simulink model "calcAcceleration"  (R2019a)
settings: Solver=FixedStepAuto  StartTime=0  StopTime=inf  FixedStep=1e-3  MaxStep=1e-3  RelTol=1e-3
values from neighbouring files (symbols this model uses):
  init =     [course_data_0_1m.mat]
libraries: simulink x1
settings Model: Creator=Frieder Uerlings  LastModifiedBy=Frieder Uerlings
settings SolverCC: ZeroCrossControl=DisableAll  AlgebraicLoopSolver=LineSearch

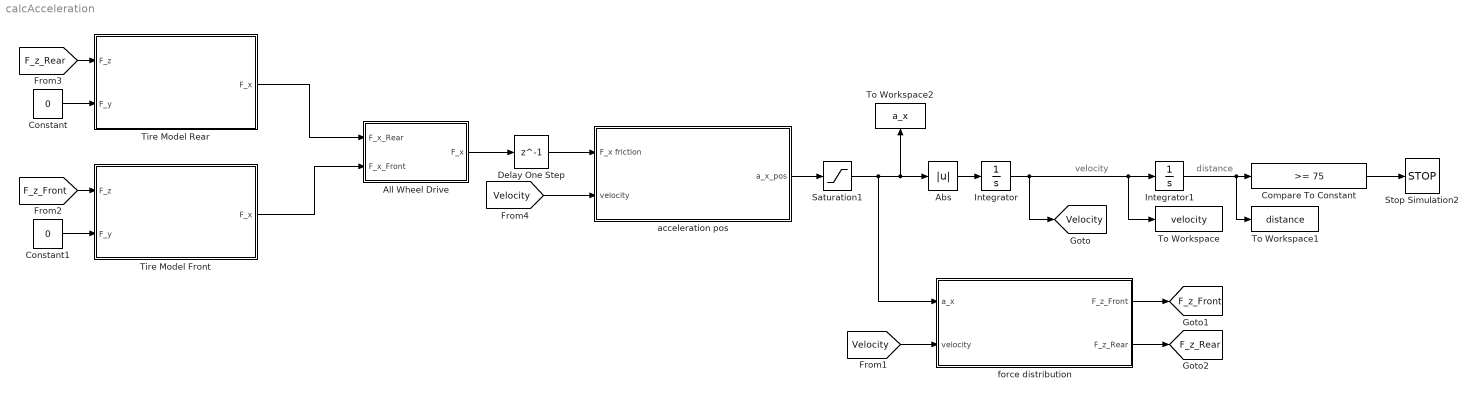
== system calcAcceleration ==
  note: distance
  note: velocity
  Abs : Abs
  All Wheel Drive : Subsystem
  Compare To Constant : simulink/Logic and Bit Operations/Compare To Constant  relop=>=  const=75  OutDataTypeStr=boolean
  Constant : Constant  Value=0
  Constant1 : Constant  Value=0
  Delay One Step : Delay  DelayLength=1
  Integrator : Integrator  InitialCondition=1/inf
  Integrator1 : Integrator
  Saturation1 : Saturate  UpperLimit=inf  LowerLimit=0  ZeroCross=off
  Stop Simulation2 : Stop
  Tire Model Front : Subsystem
  Tire Model Rear : Subsystem
  To Workspace : ToWorkspace  VariableName=velocity  SampleTime=-1
  To Workspace1 : ToWorkspace  VariableName=distance  SampleTime=-1
  To Workspace2 : ToWorkspace  VariableName=a_x  SampleTime=-1
  "acceleration pos " : Subsystem
  force distribution : Subsystem
  tag scope: F_z_Front=global, F_z_Rear=global, Velocity=global
  wires:
  Compare To Constant/1 -> Stop Simulation2/1
  Integrator/1 -> [Velocity], To Workspace/1, Integrator1/1
  Saturation1/1 -> Abs/1, To Workspace2/1, force distribution/1("a_x ")
  Integrator1/1 -> To Workspace1/1, Compare To Constant/1
  [Velocity] -> force distribution/2("velocity ")
  force distribution/1(F_z_Front) -> [F_z_Front]
  force distribution/2("F_z_Rear ") -> [F_z_Rear]
  [F_z_Front] -> Tire Model Front/1(F_z)
  [F_z_Rear] -> Tire Model Rear/1(F_z)
  Delay One Step/1 -> "acceleration pos "/1(F_x friction)
  "acceleration pos "/1("a_x_pos ") -> Saturation1/1
  Tire Model Front/1(F_x) -> All Wheel Drive/2(F_x_Front)
  Tire Model Rear/1(F_x) -> All Wheel Drive/1(F_x_Rear)
  [Velocity] -> "acceleration pos "/2(velocity)
  Abs/1 -> Integrator/1
  All Wheel Drive/1(F_x) -> Delay One Step/1
  Constant/1 -> Tire Model Rear/2(F_y)
  Constant1/1 -> Tire Model Front/2(F_y)

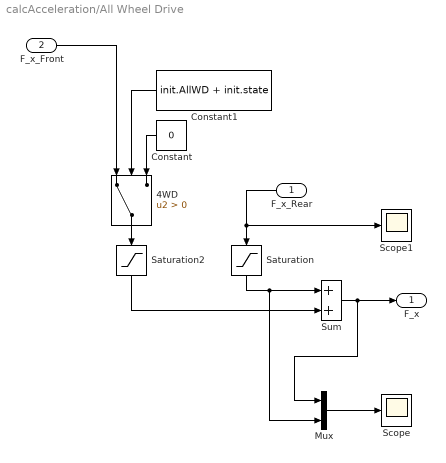
== system calcAcceleration/All Wheel Drive ==
  F_x_Rear : Inport
  F_x_Front : Inport  Port=2
  4WD : Switch  Criteria=u2 > Threshold
  Constant : Constant  Value=0
  Constant1 : Constant  Value=init.AllWD + init.state
  Mux : Mux  Inputs=2
  Saturation : Saturate  UpperLimit=inf  LowerLimit=0
  Saturation2 : Saturate  UpperLimit=inf  LowerLimit=0
  Scope : Scope
  Scope1 : Scope
  Sum : Sum
  F_x : Outport
  wires:
  Constant1/1 -> 4WD/2
  F_x_Rear/1 -> Scope1/1, Saturation/1
  4WD/1 -> Saturation2/1
  Constant/1 -> 4WD/3
  F_x_Front/1 -> 4WD/1
  Saturation/1 -> Mux/2, Sum/1
  Saturation2/1 -> Sum/2
  Sum/1 -> Mux/1, F_x/1
  Mux/1 -> Scope/1

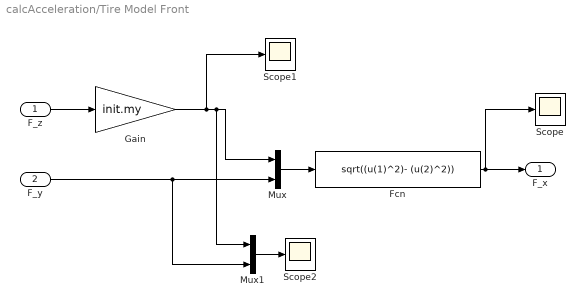
== system calcAcceleration/Tire Model Front ==
  F_z : Inport
  F_y : Inport  Port=2
  Fcn : Fcn  Expr=sqrt((u(1)^2)- (u(2)^2))
  Gain : Gain  Gain=init.my
  Mux : Mux  Inputs=2
  Mux1 : Mux  Inputs=2
  Scope : Scope
  Scope1 : Scope
  Scope2 : Scope
  F_x : Outport
  wires:
  F_z/1 -> Gain/1
  Mux/1 -> Fcn/1
  F_y/1 -> Mux1/2, Mux/2
  Fcn/1 -> Scope/1, F_x/1
  Gain/1 -> Scope1/1, Mux1/1, Mux/1
  Mux1/1 -> Scope2/1

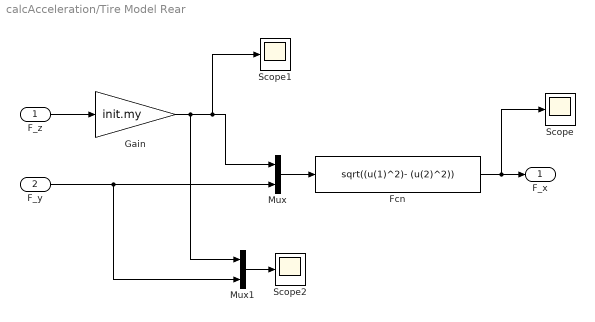
== system calcAcceleration/Tire Model Rear ==
  F_z : Inport
  F_y : Inport  Port=2
  Fcn : Fcn  Expr=sqrt((u(1)^2)- (u(2)^2))
  Gain : Gain  Gain=init.my
  Mux : Mux  Inputs=2
  Mux1 : Mux  Inputs=2
  Scope : Scope
  Scope1 : Scope
  Scope2 : Scope
  F_x : Outport
  wires:
  F_y/1 -> Mux1/2, Mux/2
  Gain/1 -> Mux1/1, Scope1/1, Mux/1
  Mux/1 -> Fcn/1
  Fcn/1 -> Scope/1, F_x/1
  F_z/1 -> Gain/1
  Mux1/1 -> Scope2/1

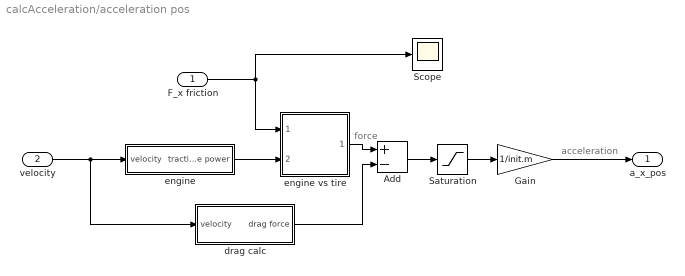
== system calcAcceleration/acceleration pos  ==
  note: force
  note: acceleration
  F_x friction : Inport
  velocity : Inport  Port=2
  Add : Sum  Inputs=+-
  Gain : Gain  Gain=1/init.m
  Saturation : Saturate  UpperLimit=inf  LowerLimit=0
  Scope : Scope
  drag calc : Subsystem
  engine : Subsystem
  engine vs tire : Subsystem
  "a_x_pos " : Outport
  wires:
  engine vs tire/1(acc force) -> Add/1
  Gain/1 -> "a_x_pos "/1
  Add/1 -> Saturation/1
  drag calc/1("drag force ") -> Add/2
  engine/1(tractive power) -> engine vs tire/2(tractive power)
  F_x friction/1 -> engine vs tire/1("a_x friction "), Scope/1
  velocity/1 -> drag calc/1(velocity), engine/1(velocity)
  Saturation/1 -> Gain/1

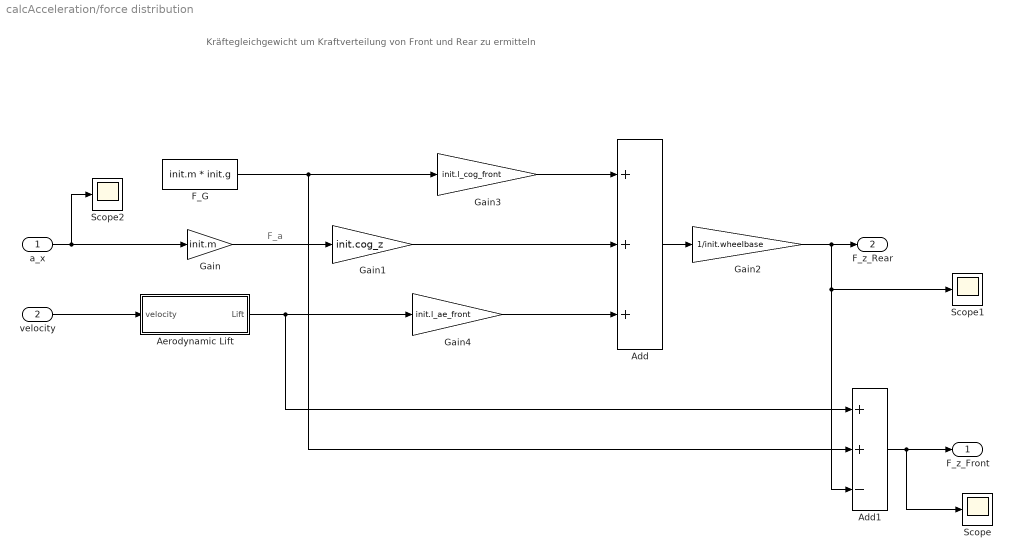
== system calcAcceleration/force distribution ==
  note: Kräftegleichgewicht um Kraftverteilung von Front und Rear zu ermitteln
  note: F_a
  "a_x " : Inport
  "velocity " : Inport  Port=2
  Add : Sum  Inputs=+++
  Add1 : Sum  Inputs=++-
  Aerodynamic Lift : Subsystem
  "F_G " : Constant  Value=init.m * init.g
  Gain : Gain  Gain=init.m
  Gain1 : Gain  Gain=init.cog_z
  Gain2 : Gain  Gain=1/init.wheelbase
  Gain3 : Gain  Gain=init.l_cog_front
  Gain4 : Gain  Gain=init.l_ae_front
  Scope : Scope
  Scope1 : Scope
  Scope2 : Scope
  F_z_Front : Outport
  "F_z_Rear " : Outport  Port=2
  wires:
  "a_x "/1 -> Scope2/1, Gain/1
  "F_G "/1 -> Add1/2, Gain3/1
  Gain3/1 -> Add/1
  Gain/1 -> Gain1/1
  "velocity "/1 -> Aerodynamic Lift/1(velocity)
  Aerodynamic Lift/1(Lift) -> Gain4/1, Add1/1
  Gain1/1 -> Add/2
  Gain4/1 -> Add/3
  Add/1 -> Gain2/1
  Gain2/1 -> Scope1/1, Add1/3, "F_z_Rear "/1
  Add1/1 -> Scope/1, F_z_Front/1

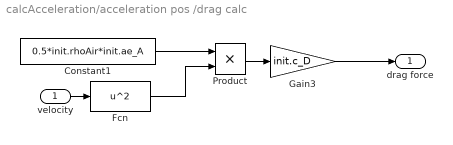
== system calcAcceleration/acceleration pos /drag calc ==
  velocity : Inport
  Constant1 : Constant  Value=0.5*init.rhoAir*init.ae_A
  Fcn : Fcn  Expr=u^2
  Gain3 : Gain  Gain=init.c_D
  Product : Product
  "drag force " : Outport
  wires:
  Constant1/1 -> Product/1
  velocity/1 -> Fcn/1
  Fcn/1 -> Product/2
  Product/1 -> Gain3/1
  Gain3/1 -> "drag force "/1

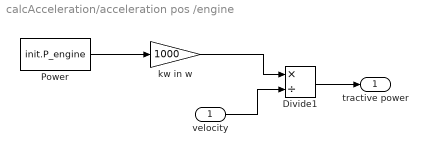
== system calcAcceleration/acceleration pos /engine ==
  velocity : Inport
  Divide1 : Product  Inputs=*/
  "Power " : Constant  Value=init.P_engine
  "kw in w " : Gain  Gain=1000
  tractive power : Outport
  wires:
  "Power "/1 -> "kw in w "/1
  "kw in w "/1 -> Divide1/1
  Divide1/1 -> tractive power/1
  velocity/1 -> Divide1/2

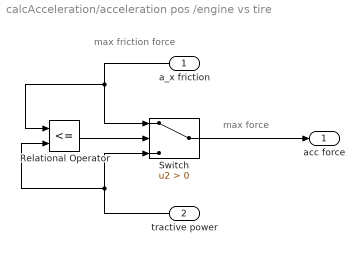
== system calcAcceleration/acceleration pos /engine vs tire ==
  note: max force
  note: max friction force
  "a_x friction " : Inport
  tractive power : Inport  Port=2
  Relational Operator : RelationalOperator  Operator=<=  OutDataTypeStr=boolean  RndMeth=Simplest
  Switch : Switch  Criteria=u2 > Threshold
  acc force : Outport
  wires:
  tractive power/1 -> Relational Operator/2, Switch/3
  "a_x friction "/1 -> Relational Operator/1, Switch/1
  Switch/1 -> acc force/1
  Relational Operator/1 -> Switch/2

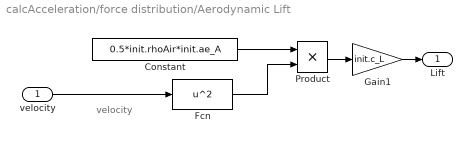
== system calcAcceleration/force distribution/Aerodynamic Lift ==
  note: velocity
  velocity : Inport
  Constant : Constant  Value=0.5*init.rhoAir*init.ae_A
  Fcn : Fcn  Expr=u^2
  Gain1 : Gain  Gain=init.c_L
  Product : Product
  Lift : Outport
  wires:
  Fcn/1 -> Product/2
  velocity/1 -> Fcn/1
  Constant/1 -> Product/1
  Product/1 -> Gain1/1
  Gain1/1 -> Lift/1
